simulink model "pendulumSIM"  (R2013b)
settings: Solver=ode45  StartTime=0.0  StopTime=10.0  MaxStep=0.05  RelTol=1e-3
undefined symbols (not defined in the file): b, g, IO, lG, M, m, theta_dot_ic, theta_ic
settings Model: Creator=richard.hill  LastModifiedBy=richard.hill

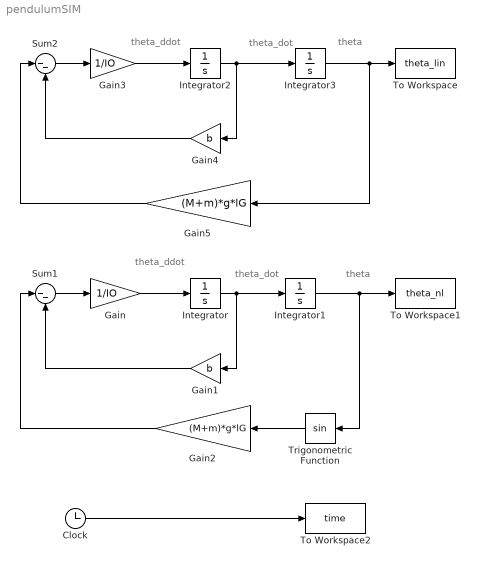
== system pendulumSIM ==
  note: theta
  note: theta_dot
  note: theta_ddot
  note: theta
  note: theta_dot
  note: theta_ddot
  Clock : Clock
  Gain : Gain  Gain=1/IO
  Gain1 : Gain  Gain=b
  Gain2 : Gain  Gain=(M+m)*g*lG
  Gain3 : Gain  Gain=1/IO
  Gain4 : Gain  Gain=b
  Gain5 : Gain  Gain=(M+m)*g*lG
  Integrator : Integrator  InitialCondition=theta_dot_ic
  Integrator1 : Integrator  InitialCondition=theta_ic
  Integrator2 : Integrator  InitialCondition=theta_dot_ic
  Integrator3 : Integrator  InitialCondition=theta_ic
  Sum1 : Sum  Inputs=|--
  Sum2 : Sum  Inputs=|--
  To Workspace : ToWorkspace  VariableName=theta_lin  SampleTime=-1
  To Workspace1 : ToWorkspace  VariableName=theta_nl  SampleTime=-1
  To Workspace2 : ToWorkspace  VariableName=time  SampleTime=-1
  Trigonometric Function : Trigonometry
  wires:
  Sum1/1 -> Gain/1
  Gain/1 -> Integrator/1
  Integrator/1 -> Gain1/1, Integrator1/1
  Integrator1/1 -> Trigonometric Function/1, To Workspace1/1
  Gain1/1 -> Sum1/2
  Trigonometric Function/1 -> Gain2/1
  Sum2/1 -> Gain3/1
  Gain3/1 -> Integrator2/1
  Integrator2/1 -> Gain4/1, Integrator3/1
  Gain4/1 -> Sum2/2
  Integrator3/1 -> Gain5/1, To Workspace/1
  Gain5/1 -> Sum2/1
  Gain2/1 -> Sum1/1
  Clock/1 -> To Workspace2/1
